simulink model "longitudinal_driver"  (R2024b)
settings: Solver=VariableStepAuto  StartTime=0.0  StopTime=10.0  RelTol=1e-3
settings Model: Creator=Loredana  LastModifiedBy=greg

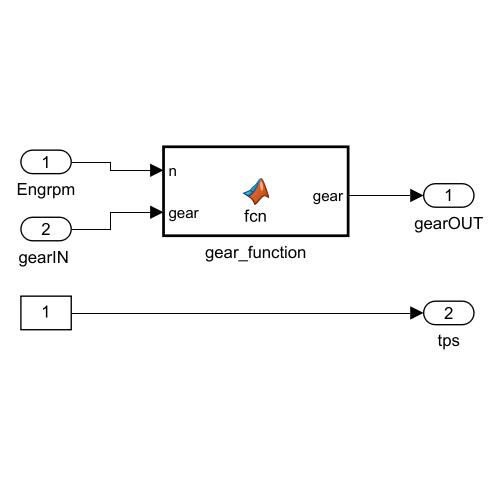
[thumbnail: Simulink's stored preview of the top-level diagram]
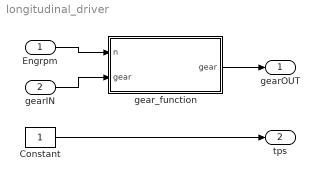
== system longitudinal_driver ==
  Engrpm : Inport
  "gearIN " : Inport  Port=2
  Constant : Constant
  gear_function : MATLAB Function  TreatAsAtomicUnit=on
  gearOUT : Outport
  tps : Outport  Port=2
  wires:
  Engrpm/1 -> gear_function/1(n)
  "gearIN "/1 -> gear_function/2("gear ")
  gear_function/1(gear) -> gearOUT/1
  Constant/1 -> tps/1

== matlab function longitudinal_driver/gear_function ==
  settings: updateMethod=CONTINUOUS
  data: n input; gear output; gear input
function gear = fcn(n, gear)
max_gear= 4;
min_gear= 2;
n_up=11000;% valore soglia massima
n_down=4000;% valore soglia minima
n_idle=4000;
   if n<=n_idle
       gear=2;   
   elseif n>n_up && gear<max_gear
        gear= gear +1;
    elseif n<n_down && gear>min_gear
        gear= gear -1;     
    end
